simulink model "CL_modelid"  (R2023a)
settings: Solver=FixedStepDiscrete  StartTime=0.0  StopTime=20  FixedStep=0.001  RelTol=1e-3  EnableMultiTasking=on
values from neighbouring files (symbols this model uses):
  amp = 1.2    [CLsweep.m]
  omega = u_ws(i)    [CLsweep.m]
undefined symbols (not defined in the file or in its folder): C, den_d, Discrete, K, num_d, sys_d, Time
libraries: quarc_library x4, ctrlSharedLib x1
settings Model: SimulationMode=external  ExtModeTrigType=signal  ExtModeTrigDuration=60000  ExtModeTrigDirection=either  ExtModeTrigLevel=0.500000  Creator=colegiusto  LastModifiedBy=colegiusto
settings SolverCC: PositivePriorityOrder=on
settings RTWCC: Description=QUARC Win64 Target Using Toolchain  SystemTargetFile=quarc_win64.tlc  Toolchain=QUARC win64 | nmake (64-bit Windows)  BuildConfiguration=Faster Runs
settings STFCustomTargetCC: TargetLangStandard=C89/C90 (ANSI)  SystemTargetFile=quarc_win64.tlc
settings GRTTargetCC: TargetLangStandard=C89/C90 (ANSI)  ParMdlRefBuildCompliant=off  CompOptLevelCompliant=off  CombineOutputUpdateFcns=off  MatFileLogging=off  CPPClassGenCompliant=off  GRTInterface=on  ExtMode=on  ExtModeMexFile=quarc_comm

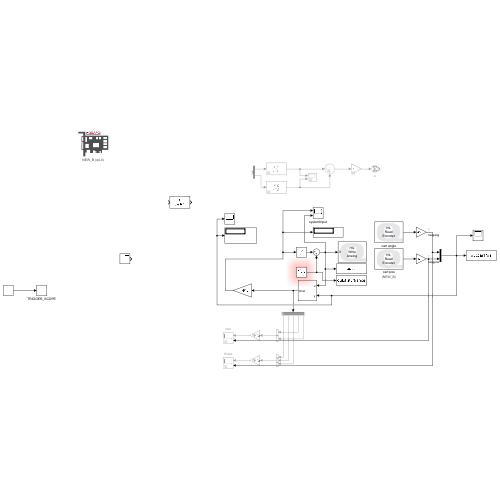
[thumbnail: Simulink's stored preview of the top-level diagram]
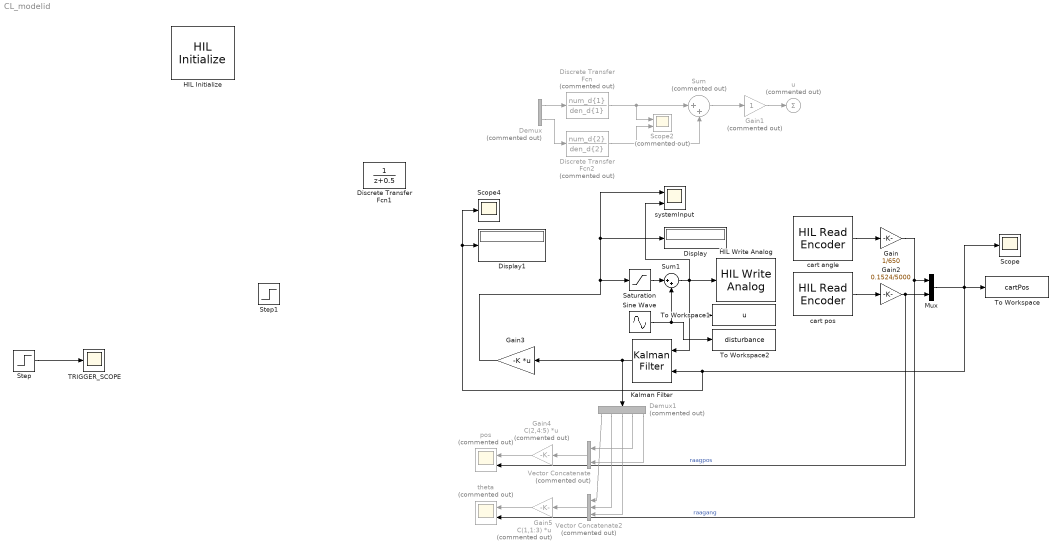
== system CL_modelid ==
  Demux : Demux  Commented=on  Outputs=2
  Demux1 : Demux  Commented=on  Outputs=5
  Discrete Transfer Fcn : DiscreteTransferFcn  Commented=on  Numerator=num_d{1}  Denominator=den_d{1}  SampleTime=0.001
  Discrete Transfer Fcn1 : DiscreteTransferFcn
  Discrete Transfer Fcn2 : DiscreteTransferFcn  Commented=on  Numerator=num_d{2}  Denominator=den_d{2}  SampleTime=0.001
  Display : Display
  Display1 : Display
  Gain : Gain  Gain=1/650
  Gain1 : Gain  Commented=on
  Gain2 : Gain  Gain=0.1524/5000
  Gain3 : Gain  Gain=-K  Multiplication=Matrix(K*u)
  Gain4 : Gain  Commented=on  Gain=C(2,4:5)  Multiplication=Matrix(K*u)
  Gain5 : Gain  Commented=on  Gain=C(1,1:3)  Multiplication=Matrix(K*u)
  HIL Initialize : quarc_library/Data Acquisition/Generic/Configuration/HIL Initialize  object_name=NEW_B  board_type=q4  board_number=0  board_options=""  exclusive=off  active=on  hardware_clocks=[0:1]  clock_modes=[0 0]  initial_clock_frequencies=[]  set_clock_params_at_start=on  set_clock_params_at_switch_in=off  set_clock_frequencies_at_start=off  set_clock_frequencies_at_switch_in=off  analog_input_channels=[0:3]  analog_input_configurations=[]  analog_input_maximums=10  analog_input_minimums=-10  set_analog_input_params_at_start=off  set_analog_input_params_at_switch_in=off  analog_output_channels=[0:3]  analog_output_maximums=[10]  analog_output_minimums=[-10]  initial_analog_outputs=[0]  final_analog_outputs=[0]  watchdog_analog_outputs=0  set_analog_output_params_at_start=on  set_analog_output_params_at_switch_in=off  set_analog_outputs_at_start=on  set_analog_outputs_at_switch_in=off  set_analog_outputs_at_terminate=on  set_analog_outputs_at_switch_out=off  set_analog_outputs_on_watchdog=off  digital_input_channels=[]  digital_output_channels=[]  digital_output_configuration=[]  initial_digital_outputs=[1]  final_digital_outputs=[1]  watchdog_digital_outputs=[2]  set_digital_output_params_at_start=off  set_digital_output_params_at_switch_in=off  set_digital_outputs_at_start=on  set_digital_outputs_at_switch_in=off  set_digital_outputs_at_terminate=on  set_digital_outputs_at_switch_out=off  set_digital_outputs_on_watchdog=off  encoder_channels=[0:3]  quadrature=[4]  encoder_filter_frequency=(1/60e-9)/1  initial_encoder_counts=[0]  set_encoder_params_at_start=on  set_encoder_params_at_switch_in=off  set_encoder_counts_at_start=on  set_encoder_counts_at_switch_in=off  pwm_channels=[]  pwm_modes=[0]  pwm_frequency=(1/60e-9)/1024  pwm_configuration=[]  pwm_alignment=[]  pwm_polarity=[]  pwm_leading_deadband=[]  pwm_trailing_deadband=[]  initial_pwm_outputs=[0]  final_pwm_outputs=[0]  watchdog_pwm_outputs=[]  set_pwm_params_at_start=on  set_pwm_params_at_switch_in=off  set_pwm_outputs_at_start=on  set_pwm_outputs_at_switch_in=off  set_pwm_outputs_at_terminate=on  set_pwm_outputs_at_switch_out=off  set_pwm_outputs_on_watchdog=off  other_output_channels=[]  initial_other_outputs=[]  final_other_outputs=[]  watchdog_other_outputs=[]  set_other_outputs_at_start=off  set_other_outputs_at_switch_in=off  set_other_outputs_at_terminate=off  set_other_outputs_at_switch_out=off  set_other_outputs_on_watchdog=off
  HIL Write Analog : quarc_library/Data Acquisition/Generic/Immediate I//O/HIL Write Analog  object_name=NEW_B  channels=0  sample_time=0.001  active=off  vector_input=off
  Kalman Filter : ctrlSharedLib/Kalman Filter  TimeDomain=Discrete-Time  UseCurrentEstimator=on  ModelSource=Individual A, B, C, D matrices  ModelSourceVariable=ss(0.95,1,1,0,1)  A=sys_d.A  B=sys_d.B  C=sys_d.C  D=sys_d.D  NumberOfStates=1  NumberOfInputs=1  NumberOfOutputs=1  InitialEstimateSource=Dialog  X0=0  P0=10  UseK=off  UseGH=off  NumberOfProcessNoiseInputs=1  G=1  TimeInvariantG=on  H=0  TimeInvariantH=on  Q=1  TimeInvariantQ=on  R=10  TimeInvariantR=on  N=0  TimeInvariantN=on  AddInputPort=on  AddEnablePort=off  OutputEstimatedY=off  OutputP=off  Ts=0.001
  Mux : Mux  Inputs=2
  Saturation : Saturate  UpperLimit=5  LowerLimit=-5
  Scope : Scope
  Scope2 : Scope  Commented=on  NumInputPorts=2
  Scope4 : Scope
  Sine Wave : Sin  Amplitude=amp  Frequency=omega  SampleTime=0.001
  Step : Step  Time=0.001  SampleTime=0
  Step1 : Step  After=0.3  SampleTime=0
  Sum : Sum  Commented=on  Inputs=|++
  Sum1 : Sum  Inputs=|++
  TRIGGER_SCOPE : Scope
  To Workspace : ToWorkspace  VariableName=cartPos  SaveFormat=Structure With Time  SampleTime=-1
  To Workspace1 : ToWorkspace  VariableName=u  SaveFormat=Structure  SampleTime=-1
  To Workspace2 : ToWorkspace  VariableName=disturbance  SaveFormat=Structure  SampleTime=-1
  Vector Concatenate : Concatenate  Commented=on
  Vector Concatenate2 : Concatenate  Commented=on  NumInputs=3
  cart angle : quarc_library/Data Acquisition/Generic/Immediate I//O/HIL Read Encoder  object_name=NEW_B  channels=3  sample_time=0.001  active=on  vector_output=on  data_type_mode=Inherit via back propagation  data_type=double
  cart pos : quarc_library/Data Acquisition/Generic/Immediate I//O/HIL Read Encoder  object_name=NEW_B  channels=2  sample_time=0.001  active=on  vector_output=on  data_type_mode=Inherit via back propagation  data_type=double
  pos : Scope  Commented=on  NumInputPorts=2
  systemInput : Scope  NumInputPorts=2
  theta : Scope  Commented=on  NumInputPorts=2
  u : Sum  Commented=on  Inputs=+
  wires:
  cart angle/1 -> Gain/1
  Step/1 -> TRIGGER_SCOPE/1
  Gain/1 -> Mux/1, theta/2  "raagang"
  Mux/1 -> Scope4/1, Display1/1, Kalman Filter/2, To Workspace/1, Scope/1
  cart pos/1 -> Gain2/1
  Gain2/1 -> Mux/2, pos/2  "raagpos"
  Demux/1 -> Discrete Transfer Fcn/1
  Demux/2 -> Discrete Transfer Fcn2/1
  Sum/1 -> Gain1/1
  Discrete Transfer Fcn2/1 -> Sum/2, Scope2/2
  Discrete Transfer Fcn/1 -> Sum/1, Scope2/1
  Gain1/1 -> u/1
  Kalman Filter/1 -> Gain3/1, Demux1/1
  Gain3/1 -> Saturation/1, Display/1, systemInput/1
  Demux1/4 -> Vector Concatenate/1
  Demux1/5 -> Vector Concatenate/2
  Vector Concatenate/1 -> Gain4/1
  Demux1/1 -> Vector Concatenate2/1
  Demux1/2 -> Vector Concatenate2/2
  Demux1/3 -> Vector Concatenate2/3
  Vector Concatenate2/1 -> Gain5/1
  Gain4/1 -> pos/1
  Gain5/1 -> theta/1
  Sum1/1 -> systemInput/2, Kalman Filter/1, To Workspace1/1, HIL Write Analog/1
  Sine Wave/1 -> To Workspace2/1, Sum1/2
  Saturation/1 -> Sum1/1
